simulink library "GreenBallTracking"  (R2016a)
settings: Solver=ode45  StartTime=0.0  StopTime=10.0  RelTol=1e-3
settings Model: Creator=sannem  LastModifiedBy=sannem
settings DataIOCC: LimitDataPoints=on
settings DebuggingCC: AllowSymbolicDim=off

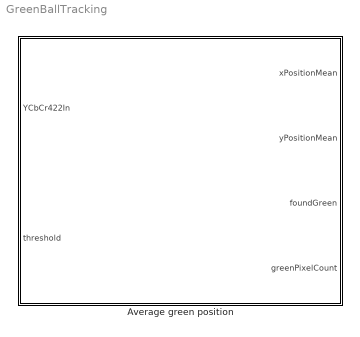
== system GreenBallTracking ==
  Average green position : MATLAB Function  TreatAsAtomicUnit=on  mask(Average green position){width=1280, height=720, downScaleFactor=4}
      mask prompts: width "Input Image width"; height "Input Image height"; downScaleFactor "Down scaling factor"
      mask help: This block returns the average x and y coordinates of all green pixels within the YCbCr 4:2:2 format input video. Specifying the downscaling factor results in the input video being downsampled by that factor in both horizontal and vertical direction to reduce computation time. The input threshold [0 - 255] controls how "green" a pixel must be before it is determined to be green

== matlab function GreenBallTracking/Average green position ==
  data: YCbCr422In input; xPositionMean output; threshold input; yPositionMean output; foundGreen output; greenPixelCount output; width parameter; height parameter; downScaleFactor parameter

function [xPositionMean, yPositionMean, foundGreen,greenPixelCount] = AverageGreenPosition(YCbCr422In,threshold,width, height, downScaleFactor)

xPosition = 0;
yPosition = 0;
xPositionMean = -1;
yPositionMean = -1;
greenPixelCount = 0;
foundGreen = 0;
inputSize = width*height*2;

c1 =     298.082/256;
Rc1 =    408.583/256;
Rc2 =   -222.921;
Gc1 =   -100.291/256;
Gc2 =   -208.120/256;
Gc3 =    135.576;
Bc1=     516.412/256;
Bc2=    -276.836;


for verticalIndex = 1 : 1 : height/downScaleFactor;             % indexing for downsampled vertical direction
    for horizontalIndex = 1 : 1 : (width / 2)/downScaleFactor;  % indexing for downsampled horizontal direction
        index = 4 * (downScaleFactor * (verticalIndex - 1) * (width / 2) + downScaleFactor * horizontalIndex) - 3;  % translate the horizontal and vertical indexes into the index into the video input
        pixel = [double(YCbCr422In(index)) double(YCbCr422In(index+1)) double(YCbCr422In(index+2)) double(YCbCr422In(index+3))];    % retrieve the pixel data and convert for calculation

        yFactor = c1 * (pixel(2)+pixel(4))/2;   % use averaging of the two chroma values for converting to RGB
        % convert to RGB and compare it with a threshold to see if its
        % green
        if (    -(yFactor + Rc1 * pixel(3) + Rc2)/2 ...  %-R/2
                -(yFactor + Bc1 * pixel(1) + Bc2)/2 ...  %-B/2
                +(yFactor + Gc1 * pixel(1) + Gc2 * pixel(3) + Gc3)...    %G
                >= threshold)

            greenPixelCount = greenPixelCount + 1;
            xPosition = xPosition + horizontalIndex * downScaleFactor;
            yPosition = yPosition + verticalIndex * downScaleFactor;
        end
    end
end
% compute the average green pixel position
if greenPixelCount > 0
    xPositionMean = 2 * xPosition / greenPixelCount;     %convert back to full width resolution
    yPositionMean = yPosition / greenPixelCount;
    foundGreen = 1;
end
end
